simulink model "massSpringDamper"  (R2016b)
settings: Solver=ode45  StartTime=0.0  StopTime=10.0  RelTol=1e-3
settings Model: Creator=alexanderhiller  LastModifiedBy=alexanderhiller
settings DataIOCC: InspectSignalLogs=on

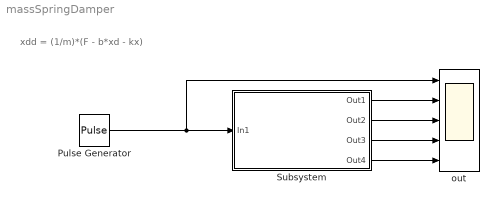
== system massSpringDamper ==
  note: xdd = (1/m)*(F - b*xd - kx)
  Pulse Generator : DiscretePulseGenerator  PulseType=Time based  Period=10  PulseWidth=5
  Subsystem : Subsystem  mask{m=10, k=0.1, b=0.1, b1=1234213, b2=23141234214}
      mask prompts: m "Mass"; k "Spring"; b "Damper"; b1 "Bloop"; b2 "Blooppp"
      mask Display: disp('Mass, spring, damper')
  out : Scope  NumInputPorts=5
  wires:
  Pulse Generator/1 -> Subsystem/1(In1), out/1
  Subsystem/1(Out1) -> out/2
  Subsystem/2(Out2) -> out/3
  Subsystem/3(Out3) -> out/4
  Subsystem/4(Out4) -> out/5

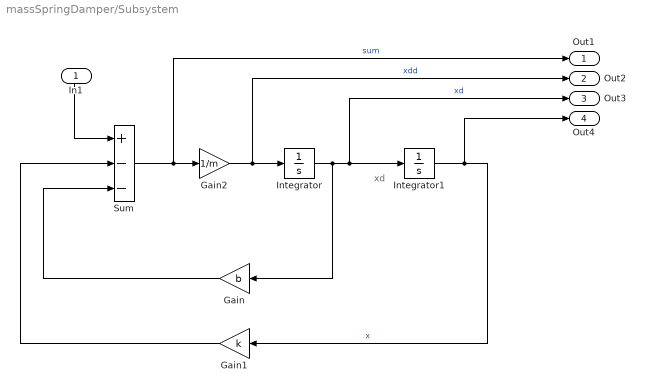
== system massSpringDamper/Subsystem ==
  note: xd
  In1 : Inport
  Gain : Gain  Gain=b
  Gain1 : Gain  Gain=k
  Gain2 : Gain  Gain=1/m
  Integrator : Integrator
  Integrator1 : Integrator
  Sum : Sum  Inputs=+--
  Out1 : Outport
  Out2 : Outport  Port=2
  Out3 : Outport  Port=3
  Out4 : Outport  Port=4
  wires:
  Integrator/1 -> Out3/1, Integrator1/1, Gain/1  "xd"
  Sum/1 -> Out1/1, Gain2/1  "sum"
  Gain/1 -> Sum/3
  Integrator1/1 -> Out4/1, Gain1/1  "x"
  Gain1/1 -> Sum/2
  Gain2/1 -> Out2/1, Integrator/1  "xdd"
  In1/1 -> Sum/1
